simulink model "diffBlocks"  (R2023b)
settings: Solver=VariableStepAuto  StartTime=0.0  StopTime=10.0  RelTol=1e-3
settings Model: Creator=neham  LastModifiedBy=neham

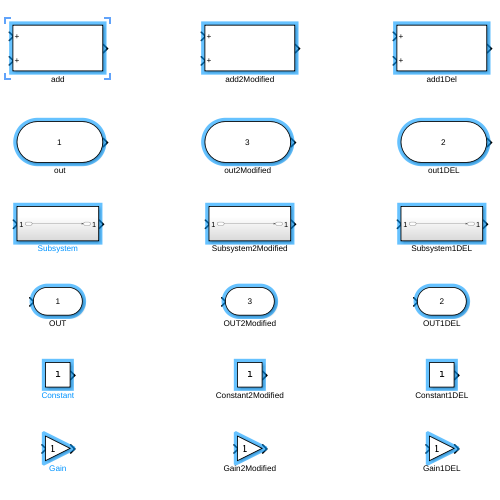
[thumbnail: Simulink's stored preview of the top-level diagram]
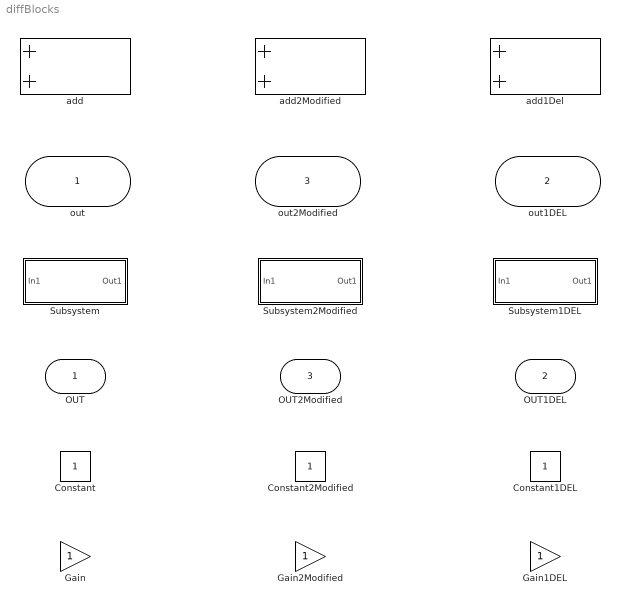
== system diffBlocks ==
  out : Inport
  out1DEL : Inport  Port=2
  out2Modified : Inport  Port=3
  Constant : Constant
  Constant1DEL : Constant
  Constant2Modified : Constant
  Gain : Gain
  Gain1DEL : Gain
  Gain2Modified : Gain
  Subsystem : Subsystem
  Subsystem1DEL : Subsystem
  Subsystem2Modified : Subsystem
  add : Sum
  add1Del : Sum
  add2Modified : Sum
  OUT : Outport
  OUT1DEL : Outport  Port=2
  OUT2Modified : Outport  Port=3

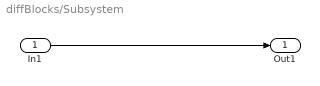
== system diffBlocks/Subsystem ==
  In1 : Inport
  Out1 : Outport
  wires:
  In1/1 -> Out1/1

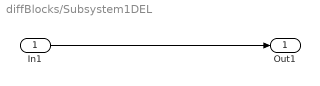
== system diffBlocks/Subsystem1DEL ==
  In1 : Inport
  Out1 : Outport
  wires:
  In1/1 -> Out1/1

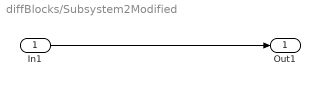
== system diffBlocks/Subsystem2Modified ==
  In1 : Inport
  Out1 : Outport
  wires:
  In1/1 -> Out1/1
